simulink model "MachCd2extensiontable"  (R2023b)
settings: Solver=VariableStepAuto  StartTime=0.0  StopTime=10.0  RelTol=1e-3
model workspace (MAT data in the model file):
  surfaceBlockParameters = Simulink.LookupTable
  surfaceBlockParameters.Table = Simulink.lookuptable.Table
  surfaceBlockParameters.Table.Value = [NaN  NaN  0.380794449822  0.728773534398  NaN  NaN  NaN  NaN  NaN  NaN; NaN  0.340919042573  0.625235126666  0.957009157245  1.00743578256  NaN  NaN  NaN  NaN  NaN; NaN  0.353129064095  0.623587727315  0.932827854759  1.01999161645  0.993209674944  1.00919848998  NaN  NaN  NaN; NaN  0.34799438672  0.580016589939  0.85209505132  1.02225906289  1.00597567868  1.02425853382  1.01771474988  NaN  NaN; NaN  0.226861582106  0.376876909549  0.518810490622  0.672066047723  0.848281603015  0.912315034914  1.01860688625  1.01252755561  NaN; NaN  0.126870515097  0.242227811563  0.341343656012  0.440732304946  0.540686733543  0.640877801771  0.74098706081  0.847669712374  0.948242976715; NaN  0.102593547356  0.219184909799  0.320129045968  0.419935690547  0.51983163298  0.619736559855  0.719639536535  0.819499251087  0.920613400955; NaN  0.126373615097  0.242999668086  0.348071164816  0.45356155619  0.558926581829  0.664568268606  0.769792885801  0.875344669256  0.984850905137; NaN  0.145349212594  0.265578858353  0.378257422798  0.491345121826  0.60466079478  0.718042208189  0.830759161789  0.945577376333  NaN; NaN  0.163436148952  0.285848572034  0.404597762166  0.523292314253  0.642106386903  0.760843310233  0.879580868316  0.998645514796  NaN]
  surfaceBlockParameters.Table.Dimensions = [10 10]
  surfaceBlockParameters.Table.DataType = 'auto'
  surfaceBlockParameters.Table.FieldName = 'Table_zData'
  surfaceBlockParameters.Breakpoints(1) = Simulink.lookuptable.Breakpoint
  surfaceBlockParameters.Breakpoints(1).Value = [0.01 0.2 0.39 0.58 0.77 0.96 1.15 1.34 1.53 1.72]
  surfaceBlockParameters.Breakpoints(1).TunableSizeName = 'N1'
  surfaceBlockParameters.Breakpoints(1).Dimensions = [1 10]
  surfaceBlockParameters.Breakpoints(1).DataType = 'auto'
  surfaceBlockParameters.Breakpoints(1).FieldName = 'BP1_xData'
  surfaceBlockParameters.Breakpoints(2) = Simulink.lookuptable.Breakpoint
  surfaceBlockParameters.Breakpoints(2).Value = [0.33 0.55 0.77 0.99 1.21 1.43 1.65 1.87 2.09 2.31]
  surfaceBlockParameters.Breakpoints(2).TunableSizeName = 'N2'
  surfaceBlockParameters.Breakpoints(2).Dimensions = [1 10]
  surfaceBlockParameters.Breakpoints(2).DataType = 'auto'
  surfaceBlockParameters.Breakpoints(2).FieldName = 'BP2_yData'
  surfaceBlockParameters.AllowMultipleInstancesOfTypeToHaveDifferentTableBreakpointSizes = 0
  surfaceBlockParameters.SupportTunableSize = 0
  surfaceBlockParameters.StructTypeInfo = Simulink.lookuptable.StructTypeInfo
  surfaceBlockParameters.StructTypeInfo.Name = 'surfaceBlockParameters_type'
  surfaceBlockParameters.StructTypeInfo.DataScope = 'Auto'
settings Model: Creator=ruotsing  LastModifiedBy=ruotsing

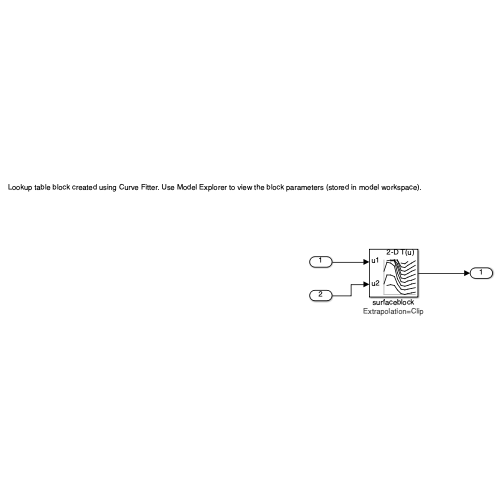
[thumbnail: Simulink's stored preview of the top-level diagram]
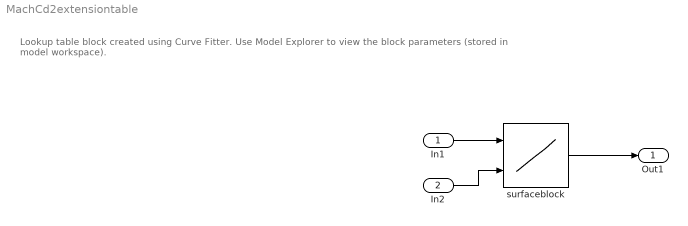
== system MachCd2extensiontable ==
  note: Lookup table block created using Curve Fitter. Use Model Explorer to view the block parameters (stored in model workspace).
  In1 : Inport
  In2 : Inport  Port=2
  surfaceblock : Lookup_n-D  DataSpecification=Lookup table object  LookupTableObject=surfaceBlockParameters  BreakpointsForDimension1=[1:3]  BreakpointsForDimension2=[1:3]  ExtrapMethod=Clip  InternalRulePriority=Speed  RndMeth=Simplest
      settings: AttributesFormatString=Extrapolation=%<ExtrapMethod>  InputPortMap=u0,u1
  Out1 : Outport
  wires:
  In2/1 -> surfaceblock/2
  surfaceblock/1 -> Out1/1
  In1/1 -> surfaceblock/1
